simulink model "task_2_2b"  (R2021b)
settings: Solver=VariableStepAuto  StartTime=0.0  StopTime=10.0  RelTol=1e-3
values from neighbouring files (symbols this model uses):
  k = 2.4716    [task_2_3.m]
  T = 0.0644    [task_2_3.m]
libraries: simulink x3
settings Model: Creator=osini  LastModifiedBy=osini

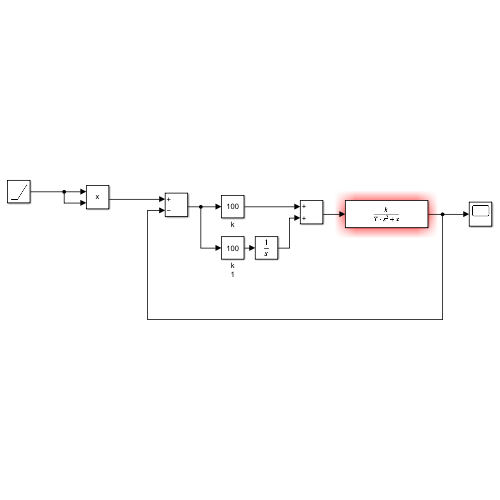
[thumbnail: Simulink's stored preview of the top-level diagram]
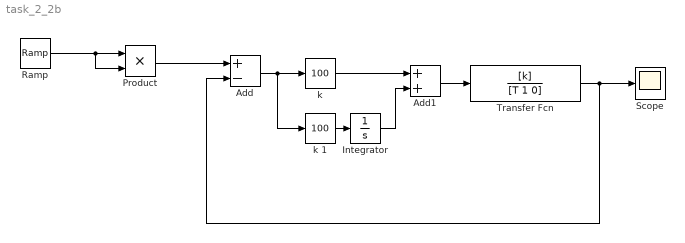
== system task_2_2b ==
  Add : Sum  Inputs=+-
  Add1 : Sum
  Integrator : Integrator
  Product : Product
  Ramp : simulink/Sources/Ramp  slope=1  start=0  InitialOutput=0
  Scope : Scope
  Transfer Fcn : TransferFcn  Numerator=[k]  Denominator=[T 1 0]
  "k " : simulink/Math Operations/Slider Gain  gain=100  low=1  high=1000
  k 1 : simulink/Math Operations/Slider Gain  gain=100  low=1  high=1000
  wires:
  Add/1 -> k 1/1, "k "/1
  Transfer Fcn/1 -> Scope/1, Add/2
  Product/1 -> Add/1
  Ramp/1 -> Product/2, Product/1
  Add1/1 -> Transfer Fcn/1
  "k "/1 -> Add1/1
  k 1/1 -> Integrator/1
  Integrator/1 -> Add1/2
